simulink model "FOC_w_LTID_linear_v3"  (R2018b)
settings: Solver=ode4  StartTime=0  StopTime=16  FixedStep=1/fs/2  MaxStep=1/fs  RelTol=1e-5  EnableMultiTasking=on
InitFcn:
  | controllers
  | model_parameters
  | KT2C = 1 / (3/2) / (Npp*Lndmpm);
  | KC2T = (3/2) * (Npp*Lndmpm);
  | Tload = 10; %ref load [Nm]
  | noise_ena = 1;
values from neighbouring files (symbols this model uses):
  B_m = 0.0016655    [model_parameters.m]
  C_m = 0.2295    [model_parameters.m]
  fs = 1*5e3    (= 5000)    [model_parameters.m]
  gamma = 0.001    [model_parameters.m]
  i_maxim_PM = 35    [model_parameters.m]
  J = 0.0146    [model_parameters.m]
  Ka_speed = 5    [controllers.m]
  Ki_id = 463    [controllers.m]
  Ki_iq = 463    [controllers.m]
  Ki_speed = 1.2    [controllers.m]
  Kp_id = 3.8    [controllers.m]
  Kp_iq = 3.8    [controllers.m]
  Kp_speed = 0.4    [controllers.m]
  Ld = 2.2e-3    (= 0.0022)    [model_parameters.m]
  Lndd_ini = Lndmpm    (= 0.12258)    [model_parameters.m]
  Lndmpm = 0.12258    [model_parameters.m]
  Lq = 2.2e-3    (= 0.0022)    [model_parameters.m]
  Npp = 4    [model_parameters.m]
  Omegae_ini = 0    [model_parameters.m]
  Rs = 0.268*1    (= 0.268)    [model_parameters.m]
  Tl_const = Trat/nrat^2    (= 6.91358024691e-07)    [model_parameters.m]
  ts = 1/fs    (= 0.0002)    [model_parameters.m]
  Vph = Vs*sqrt(2)    [model_parameters.m]
undefined symbols (not defined in the file or in its folder): d_A_e, d_A_KF, d_A_KF_col, d_B_e, d_B_KF, d_B_KF_col, d_C_e, d_C_KF, d_C_KF_col, d_D_e, d_D_KF, d_D_KF_col, DiscIntNeverNeededParam, sigbuilder_block
libraries: simulink x1
settings Model: Creator=klu  LastModifiedBy=Barna
settings DataIOCC: LimitDataPoints=on  SaveFormat=Array  SignalLoggingSaveFormat=ModelDataLogs
settings OptimizationCC: BooleanDataType=off  ExpressionDepthLimit=2147483647  InitFltsAndDblsToZero=on  LifeSpan=inf
settings DebuggingCC: AlgebraicLoopMsg=none  SaveWithParameterizedLinksMsg=none  UnderspecifiedInitializationDetection=Classic  MergeDetectMultiDrivingBlocksExec=none  SignalResolutionControl=TryResolveAllWithWarning  MultiTaskDSMMsg=warning  MultiTaskCondExecSysMsg=none  FcnCallInpInsideContextMsg=warning  StateNameClashWarn=warning  SFUnexpectedBacktrackingDiag=warning  SFNoUnconditionalDefaultTransitionDiag=warning  SFExecutionAtInitializationDiag=none
settings HardwareCC: ProdBitPerPointer=32  ProdBitPerSizeT=32  ProdBitPerPtrDiffT=32  ProdLargestAtomicFloat=None  ProdIntDivRoundTo=Undefined  ProdEndianess=Unspecified  ProdWordSize=32  ProdHWDeviceType=32-bit Generic
settings ModelReferenceCC: PropagateSignalLabelsOutOfModel=off
settings SFSimCC: SimUseLocalCustomCode=off
settings RTWCC: RTWUseLocalCustomCode=off
settings CodeAppCC: StateflowObjectComments=on
settings GRTTargetCC: TargetFcnLib=ansi_tfl_tmw.mat  TargetLangStandard=C89/C90 (ANSI)  GeneratePreprocessorConditionals=Disable all  CombineOutputUpdateFcns=off  GRTInterface=on
settings ConfigComp: CovMetricSettings=dw  CovHtmlReporting=on  CovSaveCumulativeToWorkspaceVar=on  CovSaveSingleToWorkspaceVar=on  CovExternalEMLEnable=off  CovSFcnEnable=off

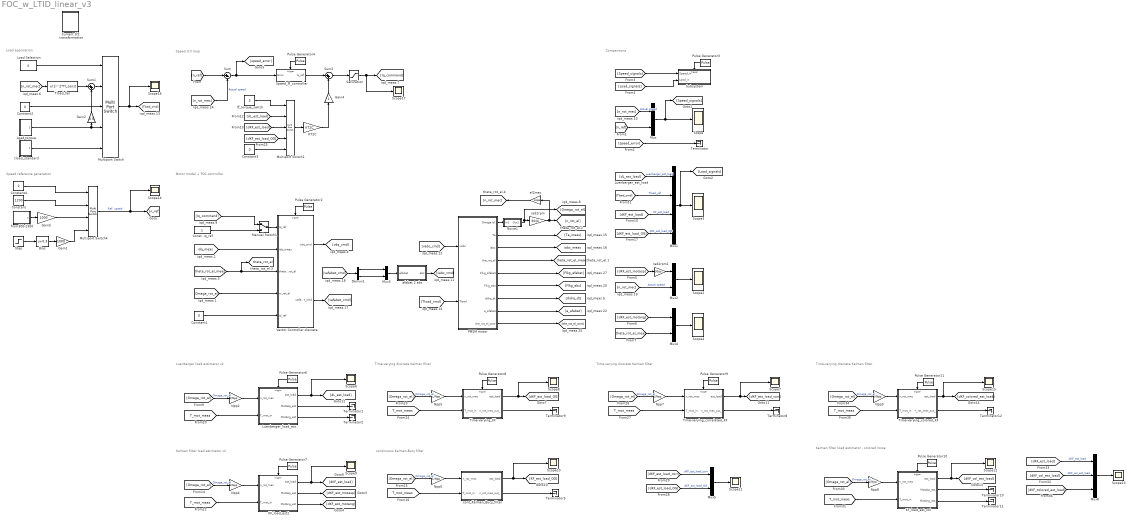
== system FOC_w_LTID_linear_v3 ==
  note: Comparisons
  note: Speed ctrl loop
  note: Speed reference generation
  note: Motor model + FOC controller
  note: Load application
  note: Luenberger load estimator v2
  note: Kalman filter load estimator v2
  note: continuous Kalman-Bucy filter
  note: Time-varying discrete Kalman filter
  note: Time-varying discrete Kalman filter
  note: Kalman filter load estimator - colored noise
  note: Time-varying discrete Kalman filter
  Bias : Bias  Bias=0.3
  Const. iq_ref : Constant
  Constant : Constant  Value=1200
  Constant1 : Constant  Value=0
  Constant2 : Constant  Value=0
  Constant3 : Constant  Value=0
  Constant4 : Constant  Value=2
  Current 3/2 transformation : Subsystem
      mask Display:
      | plot([0.1000    0.1357    0.1714    0.2071    0.2429    0.2786    0.3143    0.3500    0.3857    0.4214 0.4571    0.4929    0.5286    0.5643    0.6000]-0.05,0.4+0.6*[0.5000    0.5868    0.6564    0.6950    0.6950    0.6564    0.5868    0.5000    0.4132    0.3436 0.3050    0.3050    0.3436    0.4132    0.5000])
      | 
      | plot([0.1,0.9],[0.1,0.9])
      | 
      | plot([0.5,0.9],0.3*[1 1])
  Demux1 : Demux  Outputs=2
  Gain1 : Gain  Gain=1000
  Gain2 : Gain  Gain=0.5
  Gain4 : Gain
  Gain5 : Gain  Gain=1000
  KF_load_est2 : Subsystem
  KF_load_est_col : Subsystem
  KT2C : Gain  Gain=KT2C
  Load Selection : Constant  Value=4
  Load torque : Subsystem
  Luenberger_load_est : Subsystem
  Manual Switch1 : ManualSwitch
  Multiport Switch : MultiPortSwitch  Inputs=4
  Multiport Switch1 : MultiPortSwitch  Inputs=4
  Multiport Switch4 : MultiPortSwitch
  Mux{,2..5} (5 alike) : Mux  Inputs=2
  Mux1 : Mux
  Mux6 : Mux  Inputs=3
  Noise1 : Subsystem
  Npp{2,4..9} (7 alike) : Gain  Gain=1/Npp
  PMSM motor : Subsystem
  Pulse Generator{2..3,6..11} (8 alike) : DiscretePulseGenerator  PulseType=Time based  Period=1/fs  PulseWidth=50
  Pulse Generator4 : DiscretePulseGenerator  PulseType=Time based  Period=1/fs*1  PulseWidth=50
  Saturation : Saturate  UpperLimit=i_maxim_PM  LowerLimit=-i_maxim_PM
  Scope{,2..4,6..17} (16 alike) : Scope
  Speed_PI_controller : Subsystem
  Step : Step  SampleTime=0
  Subsystem : Subsystem
  Sum : Sum  Inputs=|+-
  Sum1 : Sum  Inputs=|++
  Sum2 : Sum  Inputs=|++
  Terminator{,1..2,5,8..12} (9 alike) : Terminator
  Time-varying_KF : Subsystem
  Time-varying_colored_KF : Subsystem
  Time-varying_correlated_KF : Subsystem
  Tload_fan : Fcn  Expr=u(1)^2*Tl_const
  Vector Controller.discrete : Subsystem
  afabet 2 abc : Subsystem
  cont_Kalman_Bucy_filter : Subsystem
  el2mec : Gain  Gain=1/Npp
  ff_torque_switch : Constant  Value=3
  "from300-1300 " : Subsystem  Tag=STV Subsys  LoadFcn=sigbuilder_block('load');  StartFcn=sigbuilder_block('start');  StopFcn=sigbuilder_block('stop');  ClipboardFcn=sigbuilder_block('clipboard');  mask(Sigbuilder block){tuvar=[0:10]}
      mask help: Sigbuilder GUI
      mask init:
      | if ~strcmp(get_param(bdroot(gcbh),'SimulationStatus'),'stopped') tuvar = sigbuilder_block('maskInit'); end
      settings: CopyFcn=sigbuilder_block('copy');  DeleteFcn=sigbuilder_block('delete');  ModelCloseFcn=sigbuilder_block('modelClose');  PreSaveFcn=sigbuilder_block('preSave');  PauseFcn=sigbuilder_block('pause')  ContinueFcn=sigbuilder_block('continue')  NameChangeFcn=sigbuilder_block('namechange');  OpenFcn=sigbuilder_block('open',[6 30 1428 681.75 ]);  CloseFcn=sigbuilder_block('close');
      mask Display: plot(0, 0, 100, 100,[2, 2, 32, 32, 2], [68, 8, 8, 68, 68],[32, 2], [38, 38], [32, 19, 2],[53, 60, 44], [32, 17, 17, 2],[16, 16, 31, 31]);txt = getActiveGroup(gcbh);text(2, 100, txt,'verticalAlignment', 'top');
  rad2rpm : Gain  Gain=30/pi
  rad2rpm1 : Gain  Gain=30/pi
  tload_standard : Subsystem
  tag scope: iabc_meas=global, theta_rot_el=global, theta_rot_el_meas=global
  wires:
  Manual Switch1/1 -> Vector Controller.discrete/1(iq_ref)
  Const. iq_ref/1 -> Manual Switch1/2
  [idq_meas] -> Vector Controller.discrete/2(idq_meas)
  Vector Controller.discrete/1(udq_cmd) -> [vdq_cmd]
  Vector Controller.discrete/2(uafabet_cmd) -> [vafabet_cmd]
  Constant2/1 -> Multiport Switch/3
  Load torque/1(T_load) -> Multiport Switch/4, Gain2/1
  Multiport Switch/1 -> Scope16/1, [Tload_cmd]
  [n_rot_mec] -> Tload_fan/1
  Load Selection/1 -> Multiport Switch/1
  Pulse Generator2/1 -> Vector Controller.discrete/Trigger
  Sum1/1 -> Multiport Switch/2
  Tload_fan/1 -> Sum1/1
  Constant1/1 -> Vector Controller.discrete/5(Id_ref)
  Gain2/1 -> Sum1/2
  PMSM motor/2(Te) -> [Te_meas]
  [vabc_cmd] -> PMSM motor/1(vabc)
  rad2rpm/1 -> el2mec/1, [n_rot_el]
  PMSM motor/4(the_rot_el) -> [theta_rot_el_meas]
  PMSM motor/5(Flkg_afabet) -> [Flkg_afabet]
  PMSM motor/6(Flkg_abc) -> [Flkg_abc]
  [Tload_cmd] -> PMSM motor/2(Tload)
  PMSM motor/3(iabc) -> [iabc_meas]
  PMSM motor/7(didiq_dt) -> [didiq_dt]
  Demux1/2 -> Mux3/2
  Demux1/1 -> Mux3/1
  [vafabet_cmd] -> Demux1/1
  afabet 2 abc/1(abc) -> [vabc_cmd]
  Mux3/1 -> afabet 2 abc/1(afabet)
  el2mec/1 -> [n_rot_mec]
  [Iq_command] -> Manual Switch1/1
  [theta_rot_el_meas] -> [theta_rot_el], Vector Controller.discrete/3(theta_rot_el)
  [Omega_rot_el] -> Vector Controller.discrete/4(w_rot_el)
  PMSM motor/8(e_afabet) -> [e_afabet]
  Multiport Switch4/1 -> Scope14/1, [n_ref]  "Ref. speed"
  Pulse Generator4/1 -> Speed_PI_controller/Trigger
  Sum/1 -> Speed_PI_controller/1(Error), [speed_error]
  Constant4/1 -> Multiport Switch4/1
  Constant/1 -> Multiport Switch4/2
  PMSM motor/9(the_rot_el_cont) -> [the_rot_el_cont]
  tload_standard/1(T_load) -> Multiport Switch/5
  "from300-1300 "/1(n) -> Gain5/1
  [n_rot_mec] -> Sum/2  "Actual speed"
  [n_ref] -> Sum/1
  Gain5/1 -> Multiport Switch4/3
  Step/1 -> Bias/1
  Bias/1 -> Gain1/1
  Gain1/1 -> Multiport Switch4/4
  Speed_PI_controller/1(iq_ref) -> Sum2/1
  Sum2/1 -> Saturation/1
  Gain4/1 -> Sum2/2
  KT2C/1 -> Gain4/1
  [Speed_signals] -> Subsystem/1(Speed_in)
  [Load_signals] -> Subsystem/2(Load_in)
  [n_ref] -> Mux/2
  [n_rot_mec] -> Mux/1  "Actual speed"
  [speed_error] -> Terminator/1
  Mux/1 -> [Speed_signals], Scope/1
  Pulse Generator3/1 -> Subsystem/Trigger
  [dL_est_load] -> Mux1/1  "Luenberger_est_load"
  Mux1/1 -> [Load_signals], Scope3/1
  [Tload_cmd] -> Mux1/2  "Tload_ref"
  [n_rot_mec] -> Mux2/2  "Actual speed"
  Mux2/1 -> Scope2/1
  [dKF_est_motasp] -> rad2rpm1/1
  rad2rpm1/1 -> Mux2/1
  [theta_rot_el_meas] -> Mux4/2
  Mux4/1 -> Scope4/1
  [dKF_est_motang] -> Mux4/1
  [Omega_rot_el] -> Npp2/1  "Omega_rot_el"
  Luenberger_load_est/3(MotAng_est) -> Terminator2/1
  Luenberger_load_est/1(est_load) -> Scope6/1, [dL_est_load]
  Npp2/1 -> Luenberger_load_est/1(n_rot_mec)
  Luenberger_load_est/2(MotAsp_est) -> Terminator1/1
  Pulse Generator6/1 -> Luenberger_load_est/Trigger
  [dKF_est_load] -> Mux1/3  "KF_est_load"
  [Omega_rot_el] -> Npp4/1  "Omega_rot_el"
  Npp4/1 -> KF_load_est2/1(n_rot_mec)
  KF_load_est2/1(est_load) -> Scope9/1, [dKF_est_load]
  Pulse Generator7/1 -> KF_load_est2/Trigger
  Multiport Switch1/1 -> KT2C/1
  ff_torque_switch/1 -> Multiport Switch1/1
  Time-varying_KF/1(est_load) -> Scope8/1, [dKF_est_load_OG]
  Pulse Generator8/1 -> Time-varying_KF/Trigger
  PMSM motor/1(Omega el.) -> Noise1/1(In1)
  [T_mot_meas] -> Luenberger_load_est/2(T_mot_in)
  [T_mot_meas] -> KF_load_est2/2(T_mot_in)
  [Omega_rot_el] -> Npp5/1  "Omega_rot_el"
  Npp5/1 -> Time-varying_KF/1(n_rot_mec)
  [T_mot_meas] -> Time-varying_KF/2(T_mot_in)
  Time-varying_KF/2(n_rot_mec_out_) -> Terminator9/1
  [dL_est_load] -> Multiport Switch1/2
  [dKF_est_load] -> Multiport Switch1/3
  [dKF_est_load_OG] -> Multiport Switch1/4
  Constant3/1 -> Multiport Switch1/5
  [T_mot_meas] -> cont_Kalman_Bucy_filter/2(T_mot_in)
  Npp6/1 -> cont_Kalman_Bucy_filter/1(n_rot_mec)
  [Omega_rot_el] -> Npp6/1  "Omega_rot_el"
  cont_Kalman_Bucy_filter/2(n_rot_mec_out_) -> Terminator5/1
  cont_Kalman_Bucy_filter/1(est_load) -> [KF_est_load_OG], Scope10/1
  [dKF_est_load_OG] -> Mux1/4  "dKF_est_load_OG"
  Pulse Generator9/1 -> Time-varying_correlated_KF/Trigger
  Npp7/1 -> Time-varying_correlated_KF/1(n_rot_mec)
  [Omega_rot_el] -> Npp7/1  "Omega_rot_el"
  Time-varying_correlated_KF/2(n_rot_mec_out_) -> Terminator8/1
  Time-varying_correlated_KF/1(est_load) -> Scope7/1, [dKF_est_load_corr]
  [T_mot_meas] -> Time-varying_correlated_KF/2(T_mot_in)
  [dKF_est_load_corr] -> Mux5/1  "dKF_est_load_corr"
  [dKF_est_load_OG] -> Mux5/2  "dKF_est_load_OG"
  [T_mot_meas] -> KF_load_est_col/2(T_mot_in)
  Npp8/1 -> KF_load_est_col/1(n_rot_mec)
  KF_load_est_col/3(MotAng_est) -> Terminator11/1
  KF_load_est_col/1(est_load) -> Scope12/1, [dKF_col_est_load]
  [Omega_rot_el] -> Npp8/1  "Omega_rot_el"
  Pulse Generator10/1 -> KF_load_est_col/Trigger
  KF_load_est_col/2(MotAsp_est) -> Terminator10/1
  Mux6/1 -> Scope13/1
  Time-varying_colored_KF/2(n_rot_mec_out_) -> Terminator12/1
  Time-varying_colored_KF/1(est_load) -> [dKF_colored_est_load], Scope15/1
  Pulse Generator11/1 -> Time-varying_colored_KF/Trigger
  [T_mot_meas] -> Time-varying_colored_KF/2(T_mot_in)
  Npp9/1 -> Time-varying_colored_KF/1(n_rot_mec)
  [Omega_rot_el] -> Npp9/1  "Omega_rot_el"
  Saturation/1 -> Scope17/1, [Iq_command]
  [dKF_col_est_load] -> Mux6/2  "dKF_col_est_load"
  [dKF_est_load] -> Mux6/1  "dKF_est_load"
  [dKF_colored_est_load] -> Mux6/3
  Mux5/1 -> Scope11/1
  Noise1/1(Out1) -> [Omega_rot_el], rad2rpm/1
  KF_load_est2/2(MotAsp_est) -> [dKF_est_motasp]
  KF_load_est2/3(MotAng_est) -> [dKF_est_motang]

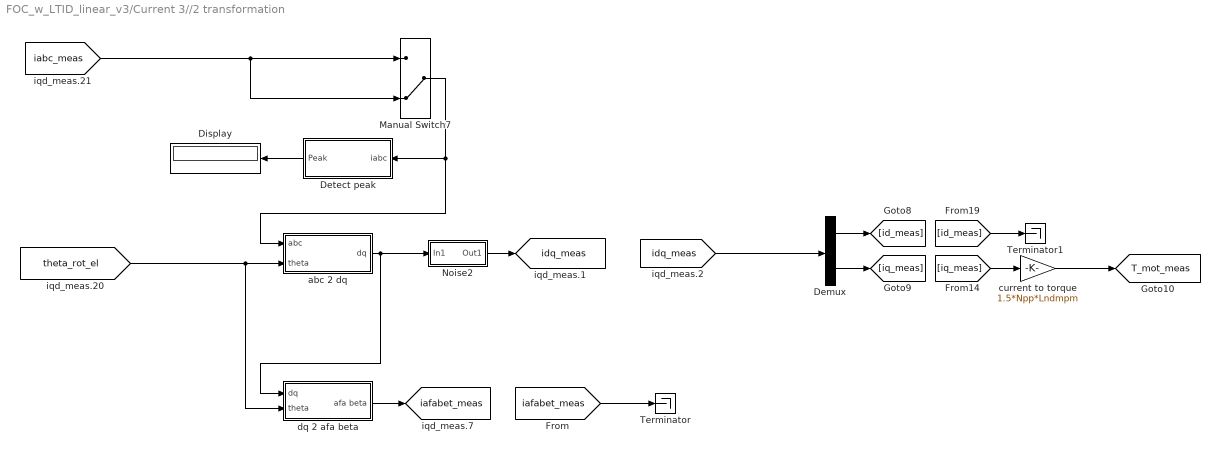
== system FOC_w_LTID_linear_v3/Current 3//2 transformation ==
  Demux : Demux  Outputs=2
  Detect peak : Subsystem
  Display : Display
  Manual Switch7 : ManualSwitch  CurrentSetting=0
  Noise2 : Subsystem
  Terminator : Terminator
  Terminator1 : Terminator
  abc 2 dq : Subsystem
  current to torque : Gain  Gain=1.5*Npp*Lndmpm
  dq 2 afa beta : Subsystem
  tag scope: T_mot_meas=global, iafabet_meas=global, idq_meas=global
  wires:
  abc 2 dq/1(dq) -> Noise2/1(In1), dq 2 afa beta/1(dq)
  dq 2 afa beta/1(afa beta) -> [iafabet_meas]
  Manual Switch7/1 -> abc 2 dq/1(abc), Detect peak/1(iabc)
  Detect peak/1(Peak) -> Display/1
  [theta_rot_el] -> abc 2 dq/2(theta), dq 2 afa beta/2(theta)
  [iabc_meas] -> Manual Switch7/1, Manual Switch7/2
  [iafabet_meas] -> Terminator/1
  Noise2/1(Out1) -> [idq_meas]
  [iq_meas] -> current to torque/1
  [idq_meas] -> Demux/1
  Demux/2 -> [iq_meas]
  current to torque/1 -> [T_mot_meas]
  [id_meas] -> Terminator1/1
  Demux/1 -> [id_meas]

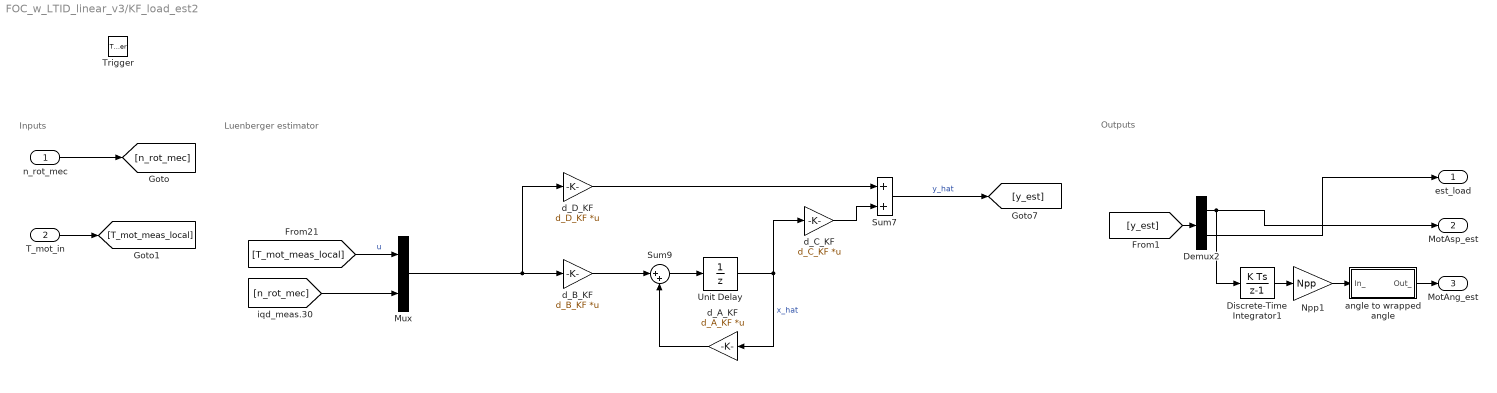
== system FOC_w_LTID_linear_v3/KF_load_est2 ==
  note: Luenberger estimator
  note: Inputs
  note: Outputs
  n_rot_mec : Inport
  T_mot_in : Inport  Port=2
  Trigger : TriggerPort  VariantControl=(inherit)
  Demux2 : Demux  Outputs=2
  Discrete-Time Integrator1 : DiscreteIntegrator  SampleTime=-1  ICPrevOutput=DiscIntNeverNeededParam  ICPrevScaledInput=DiscIntNeverNeededParam
  Mux : Mux  Inputs=2
  Npp1 : Gain  Gain=Npp
  Sum7 : Sum
  Sum9 : Sum  Inputs=|++
  Unit Delay : UnitDelay  SampleTime=-1
  angle to wrapped angle : Subsystem
  d_A_KF : Gain  Gain=d_A_KF  Multiplication=Matrix(K*u)
  d_B_KF : Gain  Gain=d_B_KF  Multiplication=Matrix(K*u)
  d_C_KF : Gain  Gain=d_C_KF  Multiplication=Matrix(K*u)
  d_D_KF : Gain  Gain=d_D_KF  Multiplication=Matrix(K*u)
  est_load : Outport
  MotAsp_est : Outport  Port=2
  MotAng_est : Outport  Port=3
  wires:
  d_B_KF/1 -> Sum9/1
  d_A_KF/1 -> Sum9/2
  Sum9/1 -> Unit Delay/1
  [n_rot_mec] -> Mux/2
  d_C_KF/1 -> Sum7/2
  Unit Delay/1 -> d_A_KF/1, d_C_KF/1  "x_hat"
  Sum7/1 -> [y_est]  "y_hat"
  Discrete-Time Integrator1/1 -> Npp1/1
  Npp1/1 -> angle to wrapped angle/1(In_)
  angle to wrapped angle/1(Out_) -> MotAng_est/1
  [T_mot_meas_local] -> Mux/1  "u"
  Mux/1 -> d_D_KF/1, d_B_KF/1
  d_D_KF/1 -> Sum7/1
  n_rot_mec/1 -> [n_rot_mec]
  T_mot_in/1 -> [T_mot_meas_local]
  [y_est] -> Demux2/1
  Demux2/2 -> est_load/1
  Demux2/1 -> Discrete-Time Integrator1/1, MotAsp_est/1

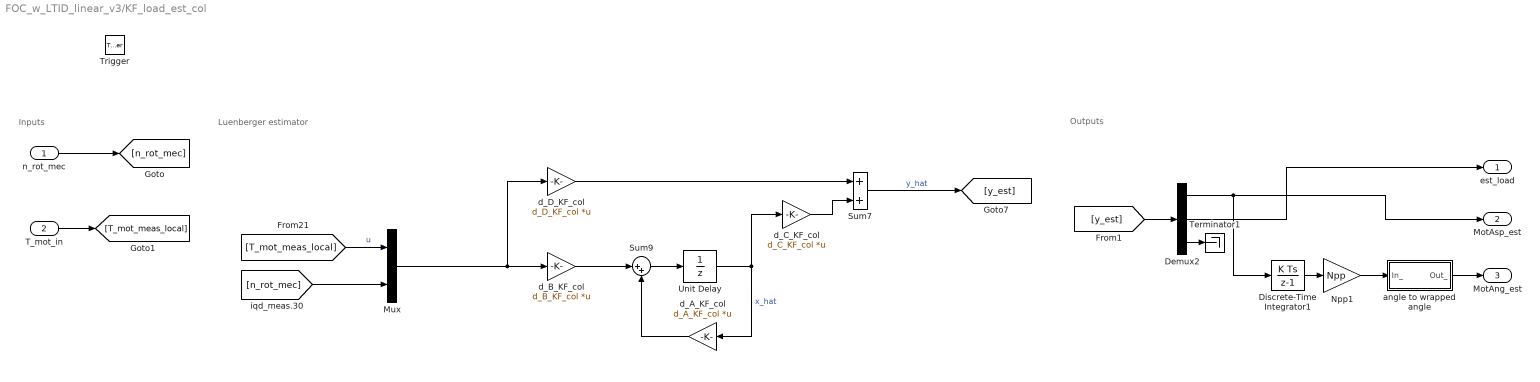
== system FOC_w_LTID_linear_v3/KF_load_est_col ==
  note: Luenberger estimator
  note: Inputs
  note: Outputs
  n_rot_mec : Inport
  T_mot_in : Inport  Port=2
  Trigger : TriggerPort  VariantControl=(inherit)
  Demux2 : Demux  Outputs=3
  Discrete-Time Integrator1 : DiscreteIntegrator  SampleTime=-1  ICPrevOutput=DiscIntNeverNeededParam  ICPrevScaledInput=DiscIntNeverNeededParam
  Mux : Mux  Inputs=2
  Npp1 : Gain  Gain=Npp
  Sum7 : Sum
  Sum9 : Sum  Inputs=|++
  Terminator1 : Terminator
  Unit Delay : UnitDelay  SampleTime=-1
  angle to wrapped angle : Subsystem
  d_A_KF_col : Gain  Gain=d_A_KF_col  Multiplication=Matrix(K*u)
  d_B_KF_col : Gain  Gain=d_B_KF_col  Multiplication=Matrix(K*u)
  d_C_KF_col : Gain  Gain=d_C_KF_col  Multiplication=Matrix(K*u)
  d_D_KF_col : Gain  Gain=d_D_KF_col  Multiplication=Matrix(K*u)
  est_load : Outport
  MotAsp_est : Outport  Port=2
  MotAng_est : Outport  Port=3
  wires:
  d_B_KF_col/1 -> Sum9/1
  d_A_KF_col/1 -> Sum9/2
  Sum9/1 -> Unit Delay/1
  [n_rot_mec] -> Mux/2
  d_C_KF_col/1 -> Sum7/2
  Unit Delay/1 -> d_A_KF_col/1, d_C_KF_col/1  "x_hat"
  Sum7/1 -> [y_est]  "y_hat"
  Discrete-Time Integrator1/1 -> Npp1/1
  Npp1/1 -> angle to wrapped angle/1(In_)
  angle to wrapped angle/1(Out_) -> MotAng_est/1
  [T_mot_meas_local] -> Mux/1  "u"
  Mux/1 -> d_D_KF_col/1, d_B_KF_col/1
  d_D_KF_col/1 -> Sum7/1
  n_rot_mec/1 -> [n_rot_mec]
  T_mot_in/1 -> [T_mot_meas_local]
  Demux2/3 -> Terminator1/1
  Demux2/2 -> est_load/1
  Demux2/1 -> Discrete-Time Integrator1/1, MotAsp_est/1
  [y_est] -> Demux2/1

== system FOC_w_LTID_linear_v3/Load torque ==
  Add : Sum  Inputs=+++
  Step Load torque 1 : Step  Time=1.5  After=Tload  SampleTime=0
  Step Load torque2 : Step  Time=2  After=-Tload  SampleTime=0
  Tload : Constant  Value=0
  T_load : Outport
  wires:
  Tload/1 -> Add/1
  Step Load torque 1/1 -> Add/2
  Step Load torque2/1 -> Add/3
  Add/1 -> T_load/1

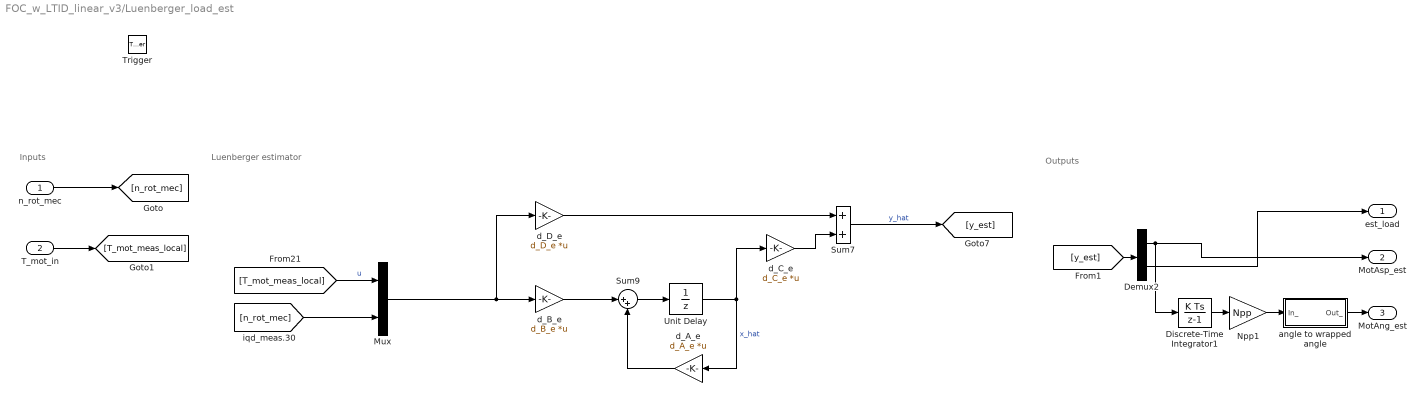
== system FOC_w_LTID_linear_v3/Luenberger_load_est ==
  note: Luenberger estimator
  note: Inputs
  note: Outputs
  n_rot_mec : Inport
  T_mot_in : Inport  Port=2
  Trigger : TriggerPort  VariantControl=(inherit)
  Demux2 : Demux  Outputs=2
  Discrete-Time Integrator1 : DiscreteIntegrator  SampleTime=-1  ICPrevOutput=DiscIntNeverNeededParam  ICPrevScaledInput=DiscIntNeverNeededParam
  Mux : Mux  Inputs=2
  Npp1 : Gain  Gain=Npp
  Sum7 : Sum
  Sum9 : Sum  Inputs=|++
  Unit Delay : UnitDelay  SampleTime=-1
  angle to wrapped angle : Subsystem
  d_A_e : Gain  Gain=d_A_e  Multiplication=Matrix(K*u)
  d_B_e : Gain  Gain=d_B_e  Multiplication=Matrix(K*u)
  d_C_e : Gain  Gain=d_C_e  Multiplication=Matrix(K*u)
  d_D_e : Gain  Gain=d_D_e  Multiplication=Matrix(K*u)
  est_load : Outport
  MotAsp_est : Outport  Port=2
  MotAng_est : Outport  Port=3
  wires:
  d_B_e/1 -> Sum9/1
  d_A_e/1 -> Sum9/2
  Sum9/1 -> Unit Delay/1
  [n_rot_mec] -> Mux/2
  d_C_e/1 -> Sum7/2
  Unit Delay/1 -> d_A_e/1, d_C_e/1  "x_hat"
  Sum7/1 -> [y_est]  "y_hat"
  n_rot_mec/1 -> [n_rot_mec]
  [T_mot_meas_local] -> Mux/1  "u"
  Mux/1 -> d_D_e/1, d_B_e/1
  d_D_e/1 -> Sum7/1
  T_mot_in/1 -> [T_mot_meas_local]
  angle to wrapped angle/1(Out_) -> MotAng_est/1
  Demux2/1 -> Discrete-Time Integrator1/1, MotAsp_est/1
  Discrete-Time Integrator1/1 -> Npp1/1
  [y_est] -> Demux2/1
  Demux2/2 -> est_load/1
  Npp1/1 -> angle to wrapped angle/1(In_)

== system FOC_w_LTID_linear_v3/Noise1 ==
  In1 : Inport
  Constant3 : Constant  Value=noise_ena
  Product2 : Product
  Random Number : RandomNumber  Variance=0.1^2  Seed=86241  SampleTime=ts/2
  Sum : Sum  Inputs=|++
  Out1 : Outport
  wires:
  In1/1 -> Sum/1
  Sum/1 -> Out1/1
  Product2/1 -> Sum/2
  Random Number/1 -> Product2/1
  Constant3/1 -> Product2/2

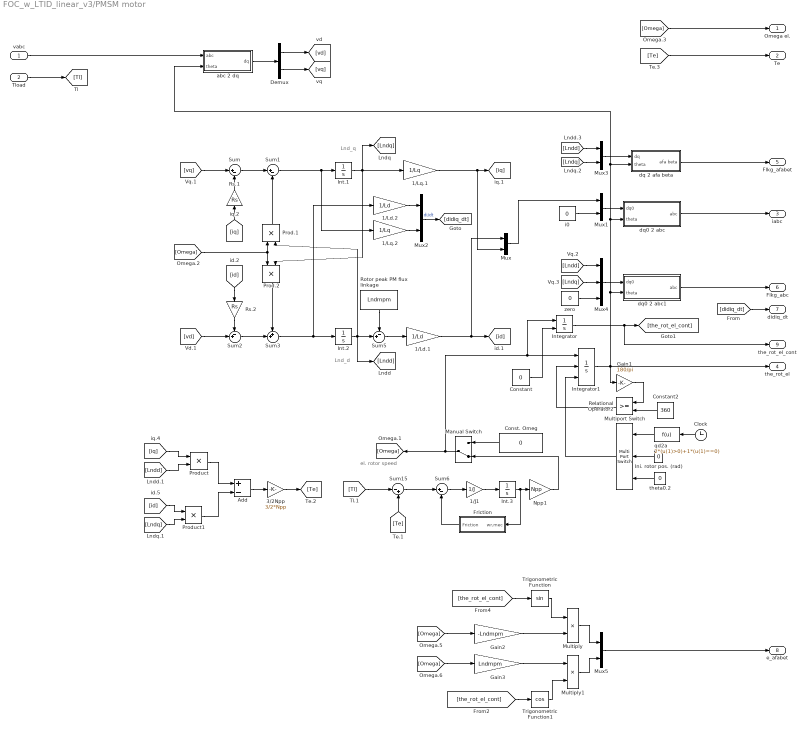
== system FOC_w_LTID_linear_v3/PMSM motor ==
  note: Lnd_d
  note: Lnd_q
  note: el. rotor speed
  vabc : Inport
  Tload : Inport  Port=2
  1/J1 : Gain  Gain=1/J
  1/Ld.1 : Gain  Gain=1/Ld
  1/Ld.2 : Gain  Gain=1/Ld
  1/Lq.1 : Gain  Gain=1/Lq
  1/Lq.2 : Gain  Gain=1/Lq
  3/2Npp : Gain  Gain=3/2*Npp
  Add : Sum  Inputs=+-
  Clock : Clock
  Const. Omeg : Constant  Value=0
  Constant : Constant  Value=0
  Constant2 : Constant  Value=360
  Demux : Demux  Outputs=2
  Friction : Subsystem
  Gain1 : Gain  Gain=180/pi
  Gain2 : Gain  Gain=-Lndmpm
  Gain3 : Gain  Gain=Lndmpm
  Ini. rotor pos. (rad) : Constant  Value=0
  Int.1 : Integrator
  Int.2 : Integrator  InitialCondition=Lndd_ini
  Int.3 : Integrator  InitialCondition=Omegae_ini/Npp
  Integrator : Integrator  InitialConditionSource=external
  Integrator1 : Integrator  ExternalReset=rising  InitialConditionSource=external  InitialCondition=pi/3
  Manual Switch : ManualSwitch  CurrentSetting=0
  Multiply : Product
  Multiply1 : Product
  Multiport Switch : MultiPortSwitch  Inputs=2
  Mux{,1..3,5} (5 alike) : Mux  Inputs=2
  Mux4 : Mux  Inputs=3
  Npp1 : Gain  Gain=Npp
  Prod.1 : Product  RndMeth=Zero
  Prod.2 : Product  RndMeth=Zero
  Product : Product  RndMeth=Zero
  Product1 : Product  RndMeth=Zero
  Relational Operator2 : RelationalOperator  OutDataTypeStr=boolean  RndMeth=Nearest
  Rotor peak PM flux linkage : Constant  Value=Lndmpm
  Rs.1 : Gain  Gain=Rs
  Rs.2 : Gain  Gain=Rs
  Sum : Sum  Inputs=|+-
  Sum1 : Sum  Inputs=|+-
  Sum15 : Sum  Inputs=|-+
  Sum2 : Sum  Inputs=-+|
  Sum3 : Sum  Inputs=++|
  Sum5 : Sum  Inputs=-+|
  Sum6 : Sum  Inputs=|+-
  Trigonometric Function : Trigonometry
  Trigonometric Function1 : Trigonometry  Operator=cos
  abc 2 dq : Subsystem
  dq 2 afa beta : Subsystem
  dq0 2 abc : Subsystem
  dq0 2 abc1 : Subsystem
  i0 : Constant  Value=0
  qd2a : Fcn  Expr=2*(u(1)>0)+1*(u(1)==0)
  theta0.2 : Constant  Value=0
  zero : Constant  Value=0
  Omega el. : Outport
  Te : Outport  Port=2
  iabc : Outport  Port=3
  the_rot_el : Outport  Port=4
  Flkg_afabet : Outport  Port=5
  Flkg_abc : Outport  Port=6
  didiq_dt : Outport  Port=7
  e_afabet : Outport  Port=8
  the_rot_el_cont : Outport  Port=9
  wires:
  3/2Npp/1 -> [Te]
  Add/1 -> 3/2Npp/1
  Sum5/1 -> 1/Ld.1/1
  Rotor peak PM flux linkage/1 -> Sum5/1
  [Te] -> Te/1
  Product1/1 -> Add/2
  Product/1 -> Add/1
  [Lndq] -> Product1/2
  [id] -> Product1/1
  [Te] -> Sum15/2
  [Tl] -> Sum15/1
  Mux/1 -> Mux1/1
  [Omega] -> Prod.2/1, Prod.1/1
  Sum3/1 -> Int.2/1, 1/Ld.2/1
  Prod.2/1 -> Sum3/1
  Sum2/1 -> Sum3/2
  [id] -> Rs.2/1
  Rs.2/1 -> Sum2/1
  [vd] -> Sum2/2
  1/Ld.1/1 -> [id], Mux/1
  Int.2/1 -> [Lndd], Sum5/2, Prod.1/2
  [iq] -> Rs.1/1
  1/Lq.1/1 -> [iq], Mux/2
  Prod.1/1 -> Sum1/2
  Sum1/1 -> Int.1/1, 1/Lq.2/1
  Int.1/1 -> 1/Lq.1/1, Prod.2/2, [Lndq]
  Sum/1 -> Sum1/1
  Rs.1/1 -> Sum/2
  [vq] -> Sum/1
  Tload/1 -> [Tl]
  Demux/2 -> [vq]
  Demux/1 -> [vd]
  i0/1 -> Mux1/2
  Mux1/1 -> dq0 2 abc/1(dq0)
  dq0 2 abc/1(abc) -> iabc/1
  vabc/1 -> abc 2 dq/1(abc)
  abc 2 dq/1(dq) -> Demux/1
  Integrator1/1 -> the_rot_el/1, dq0 2 abc/2(theta), dq 2 afa beta/2(theta), abc 2 dq/2(theta), dq0 2 abc1/2(theta), Gain1/1
  1/Ld.2/1 -> Mux2/1
  1/Lq.2/1 -> Mux2/2
  Mux3/1 -> dq 2 afa beta/1(dq)
  [Lndd] -> Mux3/1
  [Lndq] -> Mux3/2
  dq 2 afa beta/1(afa beta) -> Flkg_afabet/1
  [Lndd] -> Mux4/1
  [Lndq] -> Mux4/2
  Mux4/1 -> dq0 2 abc1/1(dq0)
  dq0 2 abc1/1(abc) -> Flkg_abc/1
  zero/1 -> Mux4/3
  Gain1/1 -> Relational Operator2/1
  Constant2/1 -> Relational Operator2/2
  [iq] -> Product/1
  [Lndd] -> Product/2
  Relational Operator2/1 -> Integrator1/2
  Ini. rotor pos. (rad)/1 -> Multiport Switch/2
  theta0.2/1 -> Multiport Switch/3
  qd2a/1 -> Multiport Switch/1
  Clock/1 -> qd2a/1
  Multiport Switch/1 -> Integrator1/3
  Const. Omeg/1 -> Manual Switch/1
  Npp1/1 -> Manual Switch/2
  Manual Switch/1 -> Integrator/1, Integrator1/1, [Omega]
  Friction/1(Friction) -> Sum6/2
  Int.3/1 -> Friction/1(wr,mec), Npp1/1
  Sum6/1 -> 1/J1/1
  1/J1/1 -> Int.3/1
  Sum15/1 -> Sum6/1
  Mux5/1 -> e_afabet/1
  Trigonometric Function1/1 -> Multiply1/2
  [Omega] -> Gain2/1
  [the_rot_el_cont] -> Trigonometric Function1/1
  Gain3/1 -> Multiply1/1
  Multiply1/1 -> Mux5/2
  [the_rot_el_cont] -> Trigonometric Function/1
  Multiply/1 -> Mux5/1
  [Omega] -> Gain3/1
  Gain2/1 -> Multiply/2
  Trigonometric Function/1 -> Multiply/1
  Integrator/1 -> the_rot_el_cont/1, [the_rot_el_cont]
  Constant/1 -> Integrator/2
  Mux2/1 -> [didiq_dt]  "di/dt"
  [didiq_dt] -> didiq_dt/1
  [Omega] -> Omega el./1

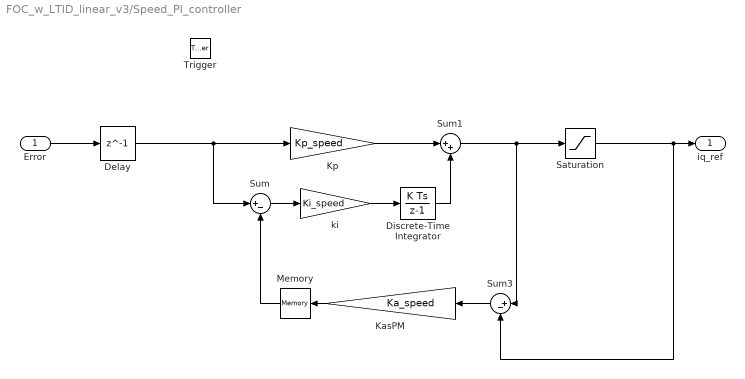
== system FOC_w_LTID_linear_v3/Speed_PI_controller ==
  Error : Inport
  Trigger : TriggerPort  VariantControl=(inherit)
  Delay : Delay  DelayLength=1
  Discrete-Time Integrator : DiscreteIntegrator  SampleTime=-1  ICPrevOutput=DiscIntNeverNeededParam  ICPrevScaledInput=DiscIntNeverNeededParam
  KasPM : Gain  Gain=Ka_speed
  Kp : Gain  Gain=Kp_speed
  Memory : Memory  InheritSampleTime=on
  Saturation : Saturate  UpperLimit=i_maxim_PM  LowerLimit=-i_maxim_PM
  Sum : Sum  Inputs=|+-
  Sum1 : Sum  Inputs=|++
  Sum3 : Sum  Inputs=|+-
  ki : Gain  Gain=Ki_speed
  iq_ref : Outport
  wires:
  Kp/1 -> Sum1/1
  ki/1 -> Discrete-Time Integrator/1
  Discrete-Time Integrator/1 -> Sum1/2
  Error/1 -> Delay/1
  KasPM/1 -> Memory/1
  Memory/1 -> Sum/2
  Sum1/1 -> Sum3/1, Saturation/1
  Sum3/1 -> KasPM/1
  Saturation/1 -> iq_ref/1, Sum3/2
  Sum/1 -> ki/1
  Delay/1 -> Sum/1, Kp/1

== system FOC_w_LTID_linear_v3/Subsystem ==
  Speed_in : Inport
  Load_in : Inport  Port=2
  Trigger : TriggerPort  VariantControl=Variant  PortDimensions=1
  To Workspace : ToWorkspace  VariableName=Speed_in  SaveFormat=Structure With Time  SampleTime=-1
  To Workspace1 : ToWorkspace  VariableName=SMO_EstLoad  SaveFormat=Structure With Time  SampleTime=-1
  wires:
  Speed_in/1 -> To Workspace/1
  Load_in/1 -> To Workspace1/1

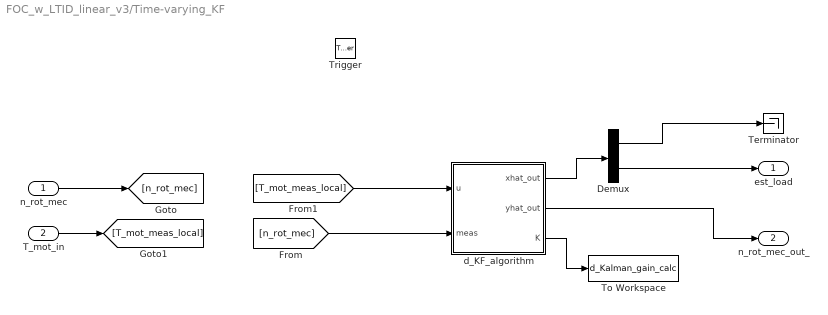
== system FOC_w_LTID_linear_v3/Time-varying_KF ==
  n_rot_mec : Inport
  T_mot_in : Inport  Port=2
  Trigger : TriggerPort  VariantControl=Variant  PortDimensions=1
  Demux : Demux  Outputs=2
  Terminator : Terminator
  To Workspace : ToWorkspace  VariableName=d_Kalman_gain_calc  SaveFormat=Structure With Time  SampleTime=-1
  d_KF_algorithm : MATLAB Function  TreatAsAtomicUnit=on
  est_load : Outport
  n_rot_mec_out_ : Outport  Port=2
  wires:
  d_KF_algorithm/3(K) -> To Workspace/1
  n_rot_mec/1 -> [n_rot_mec]
  T_mot_in/1 -> [T_mot_meas_local]
  d_KF_algorithm/2(yhat_out) -> n_rot_mec_out_/1
  d_KF_algorithm/1(xhat_out) -> Demux/1
  Demux/2 -> est_load/1
  Demux/1 -> Terminator/1
  [T_mot_meas_local] -> d_KF_algorithm/1(u)
  [n_rot_mec] -> d_KF_algorithm/2(meas)

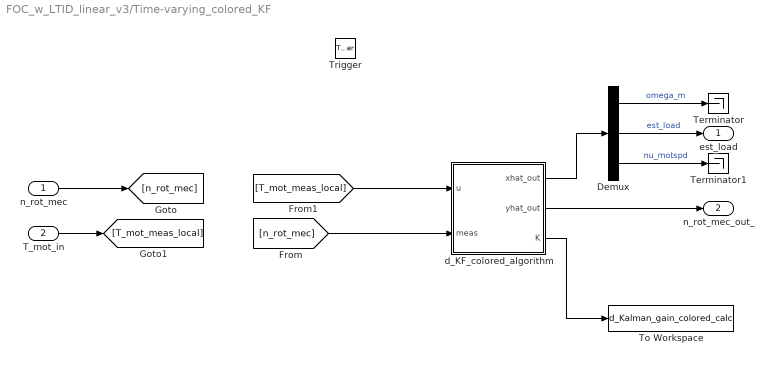
== system FOC_w_LTID_linear_v3/Time-varying_colored_KF ==
  n_rot_mec : Inport
  T_mot_in : Inport  Port=2
  Trigger : TriggerPort  VariantControl=Variant  PortDimensions=1
  Demux : Demux  Outputs=3
  Terminator : Terminator
  Terminator1 : Terminator
  To Workspace : ToWorkspace  VariableName=d_Kalman_gain_colored_calc  SaveFormat=Structure With Time  SampleTime=-1
  d_KF_colored_algorithm : MATLAB Function  TreatAsAtomicUnit=on
  est_load : Outport
  n_rot_mec_out_ : Outport  Port=2
  wires:
  d_KF_colored_algorithm/3(K) -> To Workspace/1
  n_rot_mec/1 -> [n_rot_mec]
  T_mot_in/1 -> [T_mot_meas_local]
  d_KF_colored_algorithm/1(xhat_out) -> Demux/1
  Demux/2 -> est_load/1  "est_load"
  Demux/1 -> Terminator/1  "omega_m"
  [T_mot_meas_local] -> d_KF_colored_algorithm/1(u)
  [n_rot_mec] -> d_KF_colored_algorithm/2(meas)
  Demux/3 -> Terminator1/1  "nu_motspd"
  d_KF_colored_algorithm/2(yhat_out) -> n_rot_mec_out_/1

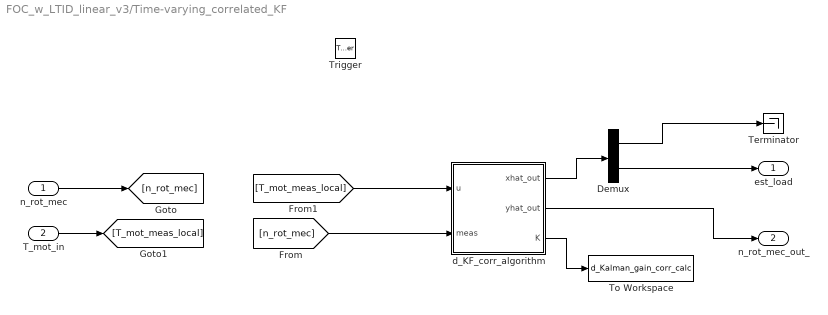
== system FOC_w_LTID_linear_v3/Time-varying_correlated_KF ==
  n_rot_mec : Inport
  T_mot_in : Inport  Port=2
  Trigger : TriggerPort  VariantControl=Variant  PortDimensions=1
  Demux : Demux  Outputs=2
  Terminator : Terminator
  To Workspace : ToWorkspace  VariableName=d_Kalman_gain_corr_calc  SaveFormat=Structure With Time  SampleTime=-1
  d_KF_corr_algorithm : MATLAB Function  TreatAsAtomicUnit=on
  est_load : Outport
  n_rot_mec_out_ : Outport  Port=2
  wires:
  d_KF_corr_algorithm/3(K) -> To Workspace/1
  n_rot_mec/1 -> [n_rot_mec]
  T_mot_in/1 -> [T_mot_meas_local]
  d_KF_corr_algorithm/2(yhat_out) -> n_rot_mec_out_/1
  d_KF_corr_algorithm/1(xhat_out) -> Demux/1
  Demux/2 -> est_load/1
  Demux/1 -> Terminator/1
  [T_mot_meas_local] -> d_KF_corr_algorithm/1(u)
  [n_rot_mec] -> d_KF_corr_algorithm/2(meas)

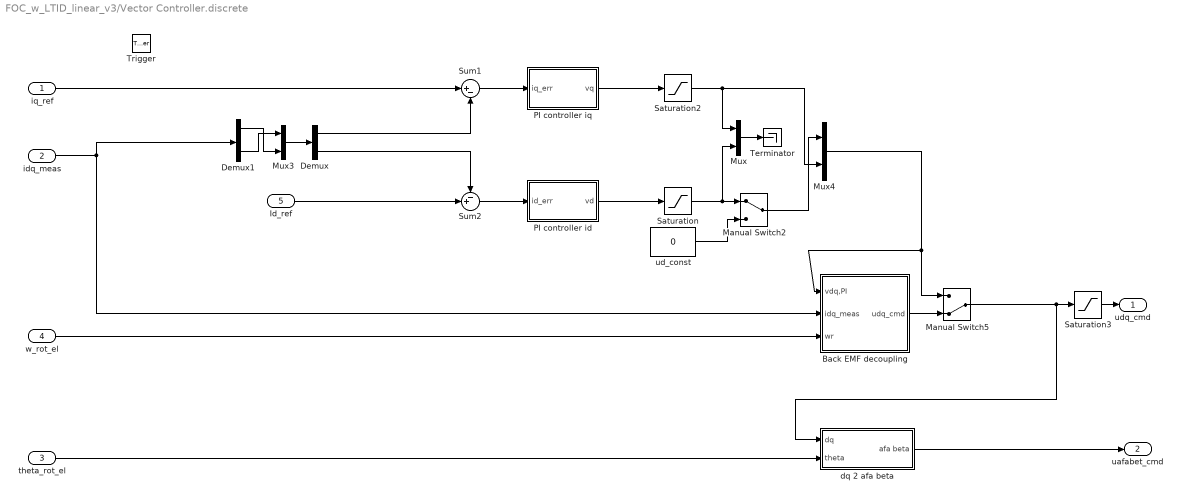
== system FOC_w_LTID_linear_v3/Vector Controller.discrete ==
  iq_ref : Inport
  idq_meas : Inport  Port=2
  theta_rot_el : Inport  Port=3
  w_rot_el : Inport  Port=4
  Id_ref : Inport  Port=5
  Trigger : TriggerPort  VariantControl=(inherit)
  Back EMF decoupling : Subsystem
  Demux : Demux  Outputs=2
  Demux1 : Demux  Outputs=2
  Manual Switch2 : ManualSwitch
  Manual Switch5 : ManualSwitch  CurrentSetting=0
  Mux : Mux  Inputs=2
  Mux3 : Mux  Inputs=2
  Mux4 : Mux  Inputs=2
  PI controller id : Subsystem
  PI controller iq : Subsystem
  Saturation : Saturate  UpperLimit=Vph  LowerLimit=-Vph
  Saturation2 : Saturate  UpperLimit=Vph  LowerLimit=-Vph
  Saturation3 : Saturate  UpperLimit=Vph  LowerLimit=-Vph
  Sum1 : Sum  Inputs=|+-
  Sum2 : Sum  Inputs=-+|
  Terminator : Terminator
  dq 2 afa beta : Subsystem
  ud_const : Constant  Value=0
  udq_cmd : Outport
  uafabet_cmd : Outport  Port=2
  wires:
  Id_ref/1 -> Sum2/2
  Saturation/1 -> Mux/2, Manual Switch2/1
  Mux/1 -> Terminator/1
  PI controller iq/1(vq) -> Saturation2/1
  Demux/1 -> Sum1/2
  PI controller id/1(vd) -> Saturation/1
  Demux/2 -> Sum2/1
  Sum1/1 -> PI controller iq/1(iq_err)
  Sum2/1 -> PI controller id/1(id_err)
  iq_ref/1 -> Sum1/1
  Saturation2/1 -> Mux/1, Mux4/2
  Manual Switch2/1 -> Mux4/1
  ud_const/1 -> Manual Switch2/2
  Demux1/2 -> Mux3/1
  Demux1/1 -> Mux3/2
  theta_rot_el/1 -> dq 2 afa beta/2(theta)
  w_rot_el/1 -> Back EMF decoupling/3(wr)
  Back EMF decoupling/1(udq_cmd) -> Manual Switch5/2
  Mux4/1 -> Manual Switch5/1, Back EMF decoupling/1(vdq,PI)
  Manual Switch5/1 -> dq 2 afa beta/1(dq), Saturation3/1
  Mux3/1 -> Demux/1
  idq_meas/1 -> Demux1/1, Back EMF decoupling/2(idq_meas)
  Saturation3/1 -> udq_cmd/1
  dq 2 afa beta/1(afa beta) -> uafabet_cmd/1

== system FOC_w_LTID_linear_v3/afabet 2 abc ==
  afabet : Inport
  Constant : Constant  Value=0
  Mux1 : Mux  Inputs=2
  Mux2 : Mux  Inputs=3
  qd2a : Fcn  Expr=u(1)+u(3)
  qd2b : Fcn  Expr=u(1)*cos(2/3*pi)+u(2)*sin(2/3*pi)+u(3)
  qd2c : Fcn  Expr=u(1)*cos(2/3*pi)-u(2)*sin(2/3*pi)+u(3)
  abc : Outport
  wires:
  Constant/1 -> Mux1/2
  qd2c/1 -> Mux2/3
  afabet/1 -> Mux1/1
  Mux1/1 -> qd2c/1, qd2b/1, qd2a/1
  qd2a/1 -> Mux2/1
  qd2b/1 -> Mux2/2
  Mux2/1 -> abc/1

== system FOC_w_LTID_linear_v3/cont_Kalman_Bucy_filter ==
  n_rot_mec : Inport
  T_mot_in : Inport  Port=2
  Demux : Demux  Outputs=2
  Integrator : Integrator
  Integrator1 : Integrator
  Terminator : Terminator
  cont_KF_algorithm : MATLAB Function  TreatAsAtomicUnit=on
  est_load : Outport
  n_rot_mec_out_ : Outport  Port=2
  wires:
  Integrator/1 -> cont_KF_algorithm/3(states_in)
  Integrator1/1 -> cont_KF_algorithm/4(P_in)
  cont_KF_algorithm/3(states_out) -> Integrator/1
  cont_KF_algorithm/4(d_P_out) -> Integrator1/1
  T_mot_in/1 -> [T_mot_meas_local]
  n_rot_mec/1 -> [n_rot_mec]
  [T_mot_meas_local] -> cont_KF_algorithm/1(u)
  [n_rot_mec] -> cont_KF_algorithm/2(meas)
  cont_KF_algorithm/2(yhat) -> n_rot_mec_out_/1
  cont_KF_algorithm/1(xhat) -> Demux/1
  Demux/2 -> est_load/1
  Demux/1 -> Terminator/1

== system FOC_w_LTID_linear_v3/from300-1300  ==
  Demux : Demux  Tag=STV Demux  Outputs=1
  FromWs : FromWorkspace  Tag=STV FromWs  VariableName=tuvar  SampleTime=0
      SigBuilderData=|
      | common.afterFinalStr = 'Extrapolate'
      | common.sampleTime = 0
      | dataSet.timeRange = [0 16]
      | dataSet.name = 'Group 1'
      | sbobj.Groups.Name = 'Group 1'
      | sbobj.Groups.Signals.Name = 'n'
      | sbobj.Groups.Signals.XData = [0 1 1.5 5 5.5 11 11.5 15 15.5 16]
      | sbobj.Groups.Signals.YData = [0.3 0.3 1.3 1.3 0.3 0.3 1.3 1.3 0.3 0.3]
      | sbobj.Groups.TimeRange = [0 16]
  n : Outport  Tag=STV Outport
  wires:
  Demux/1 -> n/1
  FromWs/1 -> Demux/1

== system FOC_w_LTID_linear_v3/tload_standard ==
  Add : Sum  Inputs=+++++
  Step Load torque 1 : Step  Time=3  After=Tload  SampleTime=0
  Step Load torque1 : Step  Time=9  After=Tload  SampleTime=0
  Step Load torque2 : Step  Time=7  After=-Tload  SampleTime=0
  Step Load torque3 : Step  Time=13  After=-Tload  SampleTime=0
  Tload_ini : Constant  Value=0
  T_load : Outport
  wires:
  Tload_ini/1 -> Add/1
  Step Load torque 1/1 -> Add/2
  Step Load torque2/1 -> Add/3
  Add/1 -> T_load/1
  Step Load torque1/1 -> Add/4
  Step Load torque3/1 -> Add/5

== system FOC_w_LTID_linear_v3/Current 3//2 transformation/Detect peak ==
  iabc : Inport
  Clock : Clock
  Compare To Constant : simulink/Logic and Bit Operations/Compare To Constant  relop=>=  const=2  OutDataTypeStr=uint8  ZeroCross=off
  Demux1 : Demux  Outputs=3
  MinMax : MinMax  Function=max  Inputs=2
  Product : Product  RndMeth=Zero
  Terminator : Terminator
  Terminator1 : Terminator
  Unit Delay : UnitDelay  SampleTime=-1
  Peak : Outport
  wires:
  iabc/1 -> Demux1/1
  Demux1/3 -> Terminator/1
  Demux1/2 -> Terminator1/1
  Clock/1 -> Compare To Constant/1
  Compare To Constant/1 -> Product/1
  Demux1/1 -> Product/2
  MinMax/1 -> Peak/1, Unit Delay/1
  Product/1 -> MinMax/1
  Unit Delay/1 -> MinMax/2

== system FOC_w_LTID_linear_v3/Current 3//2 transformation/Noise2 ==
  In1 : Inport
  Constant3 : Constant  Value=noise_ena
  Product2 : Product
  Random Number : RandomNumber  Variance=0.005^2  Seed=21874  SampleTime=ts/2
  Sum : Sum  Inputs=|++
  Out1 : Outport
  wires:
  In1/1 -> Sum/1
  Sum/1 -> Out1/1
  Product2/1 -> Sum/2
  Random Number/1 -> Product2/1
  Constant3/1 -> Product2/2

== system FOC_w_LTID_linear_v3/Current 3//2 transformation/abc 2 dq ==
  abc : Inport
  theta : Inport  Port=2
  Mux1 : Mux  Inputs=2
  Mux2 : Mux  Inputs=2
  abc2d : Fcn  Expr=2/3*(u(1)*cos(u(4))+u(2)*cos(u(4)-2*pi/3)+u(3)*cos(u(4)-4*pi/3))
  abc2q : Fcn  Expr=-1*2/3*(u(1)*sin(u(4))+u(2)*sin(u(4)-2*pi/3)+u(3)*sin(u(4)-4*pi/3))
  dq : Outport
  wires:
  Mux2/1 -> dq/1
  abc2q/1 -> Mux2/2
  abc2d/1 -> Mux2/1
  Mux1/1 -> abc2q/1, abc2d/1
  theta/1 -> Mux1/2
  abc/1 -> Mux1/1

== system FOC_w_LTID_linear_v3/Current 3//2 transformation/dq 2 afa beta ==
  dq : Inport
  theta : Inport  Port=2
  Mux1 : Mux  Inputs=2
  Mux2 : Mux  Inputs=2
  dq2afa : Fcn  Expr=u(1)*cos(u(3))-u(2)*sin(u(3))
  dq2beta : Fcn  Expr=u(1)*sin(u(3))+u(2)*cos(u(3))
  afa beta : Outport
  wires:
  dq/1 -> Mux1/1
  theta/1 -> Mux1/2
  Mux1/1 -> dq2beta/1, dq2afa/1
  dq2afa/1 -> Mux2/1
  dq2beta/1 -> Mux2/2
  Mux2/1 -> afa beta/1

== system FOC_w_LTID_linear_v3/KF_load_est2/angle to wrapped angle ==
  In_ : Inport
  Atan2 : Trigonometry  Operator=atan2
  Bias1 : Bias  Bias=-pi
  Bias2 : Bias  Bias=-pi
  Bias3 : Bias  Bias=pi
  Cos : Trigonometry  Operator=cos
  Sin : Trigonometry
  Out_ : Outport
  wires:
  Atan2/1 -> Bias3/1
  Bias1/1 -> Sin/1
  Cos/1 -> Atan2/2
  Sin/1 -> Atan2/1
  Bias2/1 -> Cos/1
  Bias3/1 -> Out_/1
  In_/1 -> Bias2/1, Bias1/1

== system FOC_w_LTID_linear_v3/KF_load_est_col/angle to wrapped angle ==
  In_ : Inport
  Atan2 : Trigonometry  Operator=atan2
  Bias1 : Bias  Bias=-pi
  Bias2 : Bias  Bias=-pi
  Bias3 : Bias  Bias=pi
  Cos : Trigonometry  Operator=cos
  Sin : Trigonometry
  Out_ : Outport
  wires:
  Atan2/1 -> Bias3/1
  Bias1/1 -> Sin/1
  Cos/1 -> Atan2/2
  Sin/1 -> Atan2/1
  Bias2/1 -> Cos/1
  Bias3/1 -> Out_/1
  In_/1 -> Bias2/1, Bias1/1

== system FOC_w_LTID_linear_v3/Luenberger_load_est/angle to wrapped angle ==
  In_ : Inport
  Atan2 : Trigonometry  Operator=atan2
  Bias1 : Bias  Bias=-pi
  Bias2 : Bias  Bias=-pi
  Bias3 : Bias  Bias=pi
  Cos : Trigonometry  Operator=cos
  Sin : Trigonometry
  Out_ : Outport
  wires:
  Atan2/1 -> Bias3/1
  Bias1/1 -> Sin/1
  Cos/1 -> Atan2/2
  Sin/1 -> Atan2/1
  Bias2/1 -> Cos/1
  Bias3/1 -> Out_/1
  In_/1 -> Bias2/1, Bias1/1

== system FOC_w_LTID_linear_v3/PMSM motor/Friction ==
  wr,mec : Inport
  Constant14 : Constant  Value=gamma
  Constant15 : Constant  Value=C_m
  Divide : Product  Inputs=*/
  Gain : Gain  Gain=0
  Gain2 : Gain  Gain=B_m
  Multiply : Product
  Sum : Sum  Inputs=|++
  Tanh : Trigonometry  Operator=tanh
  Friction : Outport
  wires:
  Divide/1 -> Tanh/1
  Tanh/1 -> Multiply/1
  Constant15/1 -> Multiply/2
  Constant14/1 -> Divide/2
  wr,mec/1 -> Divide/1, Gain2/1
  Multiply/1 -> Gain/1
  Gain2/1 -> Sum/1
  Sum/1 -> Friction/1
  Gain/1 -> Sum/2

== system FOC_w_LTID_linear_v3/PMSM motor/abc 2 dq ==
  abc : Inport
  theta : Inport  Port=2
  Mux1 : Mux  Inputs=2
  Mux2 : Mux  Inputs=2
  abc2d : Fcn  Expr=-1*2/3*(u(1)*sin(u(4))+u(2)*sin(u(4)-2*pi/3)+u(3)*sin(u(4)-4*pi/3))
  abc2q : Fcn  Expr=2/3*(u(1)*cos(u(4))+u(2)*cos(u(4)-2*pi/3)+u(3)*cos(u(4)-4*pi/3))
  dq : Outport
  wires:
  Mux2/1 -> dq/1
  abc2d/1 -> Mux2/2
  abc2q/1 -> Mux2/1
  Mux1/1 -> abc2d/1, abc2q/1
  theta/1 -> Mux1/2
  abc/1 -> Mux1/1

== system FOC_w_LTID_linear_v3/PMSM motor/dq 2 afa beta ==
  dq : Inport
  theta : Inport  Port=2
  Mux1 : Mux  Inputs=2
  Mux2 : Mux  Inputs=2
  dq2afa : Fcn  Expr=u(1)*cos(u(3))-u(2)*sin(u(3))
  dq2beta : Fcn  Expr=u(1)*sin(u(3))+u(2)*cos(u(3))
  afa beta : Outport
  wires:
  dq/1 -> Mux1/1
  theta/1 -> Mux1/2
  Mux1/1 -> dq2beta/1, dq2afa/1
  dq2afa/1 -> Mux2/1
  dq2beta/1 -> Mux2/2
  Mux2/1 -> afa beta/1

== system FOC_w_LTID_linear_v3/PMSM motor/dq0 2 abc ==
  dq0 : Inport
  theta : Inport  Port=2
  Mux1 : Mux  Inputs=2
  Mux2 : Mux  Inputs=3
  qd2a : Fcn  Expr=u(1)*cos(u(4))-u(2)*sin(u(4))+u(3)
  qd2b : Fcn  Expr=u(1)*cos(u(4)-2/3*pi)-u(2)*sin(u(4)-2/3*pi)+u(3)
  qd2c : Fcn  Expr=u(1)*cos(u(4)+2/3*pi)-u(2)*sin(u(4)+2/3*pi)+u(3)
  abc : Outport
  wires:
  Mux2/1 -> abc/1
  qd2b/1 -> Mux2/2
  qd2a/1 -> Mux2/1
  Mux1/1 -> qd2b/1, qd2c/1, qd2a/1
  theta/1 -> Mux1/2
  dq0/1 -> Mux1/1
  qd2c/1 -> Mux2/3

== system FOC_w_LTID_linear_v3/PMSM motor/dq0 2 abc1 ==
  dq0 : Inport
  theta : Inport  Port=2
  Mux1 : Mux  Inputs=2
  Mux2 : Mux  Inputs=3
  qd2a : Fcn  Expr=u(1)*cos(u(4))-u(2)*sin(u(4))+u(3)
  qd2b : Fcn  Expr=u(1)*cos(u(4)-2/3*pi)-u(2)*sin(u(4)-2/3*pi)+u(3)
  qd2c : Fcn  Expr=u(1)*cos(u(4)+2/3*pi)-u(2)*sin(u(4)+2/3*pi)+u(3)
  abc : Outport
  wires:
  qd2c/1 -> Mux2/3
  dq0/1 -> Mux1/1
  theta/1 -> Mux1/2
  Mux1/1 -> qd2a/1, qd2c/1, qd2b/1
  qd2a/1 -> Mux2/1
  qd2b/1 -> Mux2/2
  Mux2/1 -> abc/1

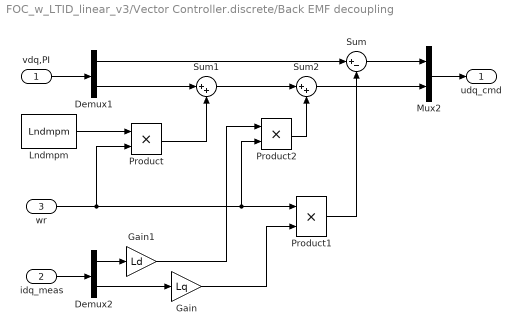
== system FOC_w_LTID_linear_v3/Vector Controller.discrete/Back EMF decoupling ==
  vdq,PI : Inport
  idq_meas : Inport  Port=2
  wr : Inport  Port=3
  Demux1 : Demux  Outputs=2
  Demux2 : Demux  Outputs=2
  Gain : Gain  Gain=Lq
  Gain1 : Gain  Gain=Ld
  Lndmpm : Constant  Value=Lndmpm
  Mux2 : Mux  Inputs=2
  Product : Product  RndMeth=Zero
  Product1 : Product  RndMeth=Zero
  Product2 : Product  RndMeth=Zero
  Sum : Sum  Inputs=|+-
  Sum1 : Sum  Inputs=|++
  Sum2 : Sum  Inputs=|++
  udq_cmd : Outport
  wires:
  Mux2/1 -> udq_cmd/1
  vdq,PI/1 -> Demux1/1
  Demux1/1 -> Sum/1
  Sum/1 -> Mux2/1
  Demux1/2 -> Sum1/1
  idq_meas/1 -> Demux2/1
  wr/1 -> Product/2, Product1/1, Product2/2
  Product1/1 -> Sum/2
  Gain/1 -> Product1/2
  Demux2/2 -> Gain/1
  Lndmpm/1 -> Product/1
  Product/1 -> Sum1/2
  Sum1/1 -> Sum2/1
  Demux2/1 -> Gain1/1
  Gain1/1 -> Product2/1
  Product2/1 -> Sum2/2
  Sum2/1 -> Mux2/2

== system FOC_w_LTID_linear_v3/Vector Controller.discrete/PI controller id ==
  id_err : Inport
  Discrete-Time Integrator : DiscreteIntegrator  SampleTime=-1  ICPrevOutput=DiscIntNeverNeededParam  ICPrevScaledInput=DiscIntNeverNeededParam
  Kp : Gain  Gain=Kp_id
  Sum1 : Sum  Inputs=|++
  ki : Gain  Gain=Ki_id
  vd : Outport
  wires:
  Sum1/1 -> vd/1
  Discrete-Time Integrator/1 -> Sum1/2
  ki/1 -> Discrete-Time Integrator/1
  Kp/1 -> Sum1/1
  id_err/1 -> ki/1, Kp/1

== system FOC_w_LTID_linear_v3/Vector Controller.discrete/PI controller iq ==
  iq_err : Inport
  Discrete-Time Integrator : DiscreteIntegrator  SampleTime=-1  ICPrevOutput=DiscIntNeverNeededParam  ICPrevScaledInput=DiscIntNeverNeededParam
  Kp : Gain  Gain=Kp_iq
  Sum1 : Sum  Inputs=|++
  ki : Gain  Gain=Ki_iq
  vq : Outport
  wires:
  Sum1/1 -> vq/1
  Discrete-Time Integrator/1 -> Sum1/2
  ki/1 -> Discrete-Time Integrator/1
  Kp/1 -> Sum1/1
  iq_err/1 -> ki/1, Kp/1

== system FOC_w_LTID_linear_v3/Vector Controller.discrete/dq 2 afa beta ==
  dq : Inport
  theta : Inport  Port=2
  Mux1 : Mux  Inputs=2
  Mux2 : Mux  Inputs=2
  dq2afa : Fcn  Expr=u(1)*cos(u(3))-u(2)*sin(u(3))
  dq2beta : Fcn  Expr=u(1)*sin(u(3))+u(2)*cos(u(3))
  afa beta : Outport
  wires:
  Mux2/1 -> afa beta/1
  dq2beta/1 -> Mux2/2
  dq2afa/1 -> Mux2/1
  Mux1/1 -> dq2afa/1, dq2beta/1
  theta/1 -> Mux1/2
  dq/1 -> Mux1/1

== matlab function FOC_w_LTID_linear_v3/Time-varying_correlated_KF/d_KF_corr_algorithm ==
  data: u input; xhat_out output; meas input; yhat_out output; K output
function [xhat_out, yhat_out, K] = fcn(u, meas)
% Time-varying discrete Kalman filter
% Correlated process and measurement noise
% x_k = A x_{k-1} B u_{k-1} + w_{k-1}
% y = C x_k + v
% x = [ omega_m, T_load ];
% u = [ T_mot ];
% w = [ omega_m, T_load ];
% y = [ omega_m ]
% Process noise
q_omega = 1/24^2; %1/36^2
q_load = 1/36^2;   %1/2^2
% Measurement noise
r_omega = 1/50^2; %1/200^2

persistent P xhat A B C D Q R M
%Initialization
if isempty(P)
    A = [  0.999977185191769  -0.013698472500730
        0   0.999999800000020];
    B = [ 0.013698473870582
        0];
    C = [ 1     0];
    D = [ 0 ];
    Q = diag([q_omega q_load]);
    R = diag([r_omega]);
    M = [-5e-4; 0];
    xhat = zeros(size(A,1), 1);
    P = zeros(size(A,1));
end
% Propagate the state estimate and covariance matrix:
% Priori state estimate
xhat = A*xhat + B*u;
P = A*P*A' + Q;
% Calculate the Kalman gain
K = (P*C'+M)/(C*P*C' + C*M + M'*C' + R);
% Calculate the measurement residual
resid = meas - (C*xhat + D*u);
% Update the state and error covariance estimate
% Posteriori state estimate
xhat = xhat + K*resid;
P = P - K*(C*P + M');
% P = (eye(size(K,1))-K*C)*P;
% Post the results
xhat_out = xhat;
yhat_out = C*xhat_out + D*u;
end

== matlab function FOC_w_LTID_linear_v3/Time-varying_colored_KF/d_KF_colored_algorithm ==
  data: u input; xhat_out output; meas input; yhat_out output; K output
function [xhat_out, yhat_out, K] = fcn(u, meas)
% Time-varying discrete Kalman filter
% With colored measurement (pink) noise
% x_k = A x_{k-1} B u_{k-1} + w_{k-1}
% y = C x_k + v
% x = [ omega_m, T_load, \nu_motspd ];
% u = [ T_mot ];
% w = [ omega_m, T_load, \zeta ];
% y = [ omega_m; \nu_motspd ]
% Process noise
q_omega = 1/24^2; %1/36^2
q_load = 1/36^2;   %1/2^2
q_omega_process = q_omega * 10^4;
% Measurement noise
r_omega = 1/50^2; %1/50^2 %1/200^2
r_omega_mod = 1e-7;

persistent P xhat A B C D Q R
%Initialization
if isempty(P)
    A = [ 0.999977185191769  -0.013698472500730                   0
        0   0.999999800000020                   0
        0                   0   0.716531310573789];
    B = [  0.013698473870582
        0
        0 ];
    C = [ 1     0     1 ];
    D = [ 0 ];
    Q = diag([q_omega q_load q_omega_process]);
    R = diag([r_omega_mod]);
    xhat = zeros(size(A,1), 1);
    P = zeros(size(A,1));
end
% Propagate the state estimate and covariance matrix:
% Priori state estimate
xhat = A*xhat + B*u;
P = A*P*A' + Q;
% Calculate the Kalman gain
K = P*C'/(C*P*C' + R);
% Calculate the measurement residual
resid = meas - (C*xhat + D*u);
% Update the state and error covariance estimate
% Posteriori state estimate
xhat = xhat + K*resid;
P = (eye(size(K,1))-K*C)*P;
% Post the results
xhat_out = xhat;
yhat_out = C*xhat_out + D*u;
end

== matlab function FOC_w_LTID_linear_v3/Time-varying_KF/d_KF_algorithm ==
  data: u input; xhat_out output; meas input; yhat_out output; K output
function [xhat_out, yhat_out, K] = fcn(u, meas)
% Time-varying discrete Kalman filter
% x_k = A x_{k-1} B u_{k-1} + w_{k-1}
% y = C x_k + v
% x = [ omega_m, T_load ];
% u = [ T_mot ];
% w = [ omega_m, T_load ];
% y = [ omega_m ]
% Process noise
q_omega = 1/24^2; %1/36^2
q_load = 1/36^2;   %1/2^2
% Measurement noise
r_omega = 1/50^2; %1/200^2

persistent P xhat A B C D Q R
%Initialization
if isempty(P)
    A = [  0.999977185191768  -0.013698472501329
        0   0.999999800000020];
    B = [ 0.013698473871176
        0];
    C = [ 0.999988592595884  -0.006849236250665 ];
    D = [ 0.006849236935588 ];
    Q = diag([q_omega q_load]);
    R = diag([r_omega]);
    xhat = zeros(size(A,1), 1);
    P = zeros(size(A,1));
end
% Propagate the state estimate and covariance matrix:
% Priori state estimate
xhat = A*xhat + B*u;
P = A*P*A' + Q;
% Calculate the Kalman gain
K = P*C'/(C*P*C' + R);
% Calculate the measurement residual
resid = meas - (C*xhat + D*u);
% Update the state and error covariance estimate
% Posteriori state estimate
xhat = xhat + K*resid;
P = (eye(size(K,1))-K*C)*P;
% Post the results
xhat_out = xhat;
yhat_out = C*xhat_out + D*u;
end

== matlab function FOC_w_LTID_linear_v3/cont_Kalman_Bucy_filter/cont_KF_algorithm ==
  data: u input; xhat output; meas input; yhat output; states_out output; states_in input; P_in input; d_P_out output
function [xhat, yhat, states_out, d_P_out] = fcn(u, meas, states_in, P_in)
% Time-varying Kalman filter
% d_x = Ax + Bu + Gw
% y = Cx + Du + v
% x = [ omega_m, T_load ]
% u = [ T_mot ]
% w = [ omega_m, T_load ]
% y = [ omega_m ]
% Tuning parameters
% Process noise
q_omega = 1/36^2; %1/36^2
q_load = 1/10^2;   %1/2^2
% Measurement noise
r_omega = 1/100^2; %1/200^2

%Initialization
 A = [ -0.1141  -68.4932
            0   -0.0010];
        B = [ 68.4932
            0];
        C = [ 1     0];
        D = [ 0 ];
        
Q = diag([q_omega q_load]);
R = diag([r_omega]);

xhat = zeros(size(A,1), 1);
yhat = zeros(size(C,1), 1);
states_out = zeros(size(A,1), 1); %#ok
d_P_out = zeros(size(A,1));

% Propagate the state estimate and covariance matrix:
% Priori state estimate
xhat = states_in;
P = P_in;
% Calculate the measurement residual
resid = meas - C*xhat;
% Calculate the filter gain
K =(P*C')/R;
% state update equations
d_xhat = A*xhat + B*u + K*resid;
d_P = A*P +P*A' - K*R*K' + Q;
% Post the results
xhat = xhat;
yhat = C*xhat;
states_out = d_xhat;
d_P_out = d_P;
end
